simulink model "SEAMOUR_Sim"  (R2023a)
settings: Solver=ode4  StartTime=0.0  StopTime=12  FixedStep=simulation_ts  MaxStep=0.001  MinStep=0.0001  RelTol=1e-3  EnableMultiTasking=on
values from neighbouring files (symbols this model uses):
  Area_y = [0.0031581,0.024875,0.025026,0.021123,0.021123,0.025026,0.024875,0.037486]    [init_file.m]
  Area_z = [0.0031588,0.028932,0.035488,0.030129,0.030129,0.035488,0.028932,0.039984]    [init_file.m]
  Cd_y = [0.5645,0.5232,0.4085,0.3589,0.3589,0.40849,0.5232,0.4642]    [init_file.m]
  Cd_z = [0.5645,0.52,0.5843,0.533,0.533,0.5843,0.52,0.5238]    [init_file.m]
  Coeff = [xudot, yvdot, zwdot]    [init_file.m]
  gravity = 9.81    [init_file.m]
  m = (4*pi*rho*a*b*b)/3    (= 16.3133743522)    [init_file.m]
  offset = 0.002    [init_file.m]
  percent_y = Area_y/t_y    [init_file.m]
  percent_z = Area_z/t_z    [init_file.m]
  xudot = k1*m    [init_file.m]
undefined symbols (not defined in the file or in its folder): center_body, headmain, headmotorshield, headmount, hindconnection, hindcover, kx_lower, kx_upper, kz_lower, kz_upper, lefthindflipper, lefthindmotor, leftmotor1, leftmotor2, leftmotor3, lf_lower, lf_upper, rf_lower, rf_upper, righthindflipper, righthindmotor, rightmotor1, rightmotor2, rightmotor3, tailmotorshield, tailmount, X, Y, Z
libraries: nesl_utility x208, sm_lib x149
(part 5 of 7)

== system SEAMOUR_Sim/Sealion Robot/Distributed Forces/Distbuted Load In y and z directions/Subsystem1 ==
  Add10 : Sum
  Add11 : Sum
  Added Mass F : MATLAB Function  TreatAsAtomicUnit=on
  Body F : sm_lib/Frames and Transforms/Rigid Transform  TranslationMethod=Cartesian  TranslationStandardOffset=0  TranslationStandardOffsetUnits=m  TranslationStandardAxis=+Z  TranslationCartesianOffset=[0.09 0 0]  TranslationCartesianOffsetUnits=m  TranslationROffset=0  TranslationROffsetUnits=m  TranslationZOffset=0  TranslationZOffsetUnits=m  TranslationThetaOffset=0  TranslationThetaOffsetUnits=deg  RotationMethod=StandardAxis  RotationAngleUnits=deg  RotationStandardAxis=+X  RotationAngle=0  RotationArbitraryAxis=[0 0 1]  FollAlignAxisA=+X  BaseAlignAxisA=+Y  FollAlignAxisB=+Y  BaseAlignAxisB=+Z  RotationSequenceAxes=FollowerAxes  RotationSequence=XYX  RotationSequenceAngles=[0 0 0]  RotationSequenceAnglesUnits=deg  RotationMatrix=[1 0 0; 0 1 0; 0 0 1]  Quaternion=[1 0 0 0]
  Constant1 : Constant  Value=Cd_z
  Constant2 : Constant  Value=Area_z
  Constant25 : Constant  Value=Cd_y
  Constant26 : Constant  Value=Area_y
  Constant28 : Constant  Value=percent_y
  Constant29 : Constant  Value=Coeff
  Constant3 : Constant  Value=percent_z
  Drag F : MATLAB Function  TreatAsAtomicUnit=on
  External Force and Torque5 : sm_lib/Forces and Torques/External Force and Torque  ForceResolutionFrame=AttachedFrame  EnableForceX=off  EnableForceY=on  EnableForceZ=on  EnableForce=off  TorqueResolutionFrame=AttachedFrame  EnableTorqueX=off  EnableTorqueY=off  EnableTorqueZ=off  EnableTorque=off
  PS-Simulink Converter{28..29,42..43} (4 alike) : nesl_utility/PS-Simulink Converter  PhysicalDomain=network_engine_domain  SubClassName=ps_output  LeftPortType=input  RightPortType=output  PseudoPeriodic=off  Frequencies=[]  VectorFormat=1-D array  Unit=1  AffineConversion=off
  Scope : Scope
  Scope1 : Scope
  Simulink-PS Converter11 : nesl_utility/Simulink-PS Converter  PhysicalDomain=network_engine_domain  SubClassName=ps_input  LeftPortType=input  RightPortType=output  PseudoPeriodic=off  Frequencies=[]  NoiseDistribution=none  NoiseParameters=[]  Unit=1  AffineConversion=off  FilteringAndDerivatives=filter  SimscapeFilterOrder=2  InputFilterTimeConstant=0.001  UdotUserProvided=0
  Simulink-PS Converter12 : nesl_utility/Simulink-PS Converter  PhysicalDomain=network_engine_domain  SubClassName=ps_input  LeftPortType=input  RightPortType=output  PseudoPeriodic=off  Frequencies=[]  NoiseDistribution=none  NoiseParameters=[]  Unit=1  AffineConversion=off  FilteringAndDerivatives=filter  SimscapeFilterOrder=2  InputFilterTimeConstant=0.001  UdotUserProvided=0
  Transfer Fcn : TransferFcn  Denominator=[0.1 1]
  Transfer Fcn1 : TransferFcn  Denominator=[0.1 1]
  Transform Sensor5 : sm_lib/Frames and Transforms/Transform Sensor  MeasurementFrame=NonRotatingFollower  RotationSequence=XYX  SenseAngle=off  SenseAxis=off  SenseQ=off  SenseR=off  SenseRotationSequence=off  SenseOmegaX=off  SenseOmegaY=off  SenseOmegaZ=off  SenseQDot=off  SenseRDot=off  SenseRotationSequenceDot=off  SenseAlphaX=off  SenseAlphaY=off  SenseAlphaZ=off  SenseQDDot=off  SenseRDDot=off  SenseX=off  SenseY=off  SenseZ=off  SenseRad=off  SenseAzim=off  SenseDist=off  SenseInc=off  SenseXDot=off  SenseYDot=on  SenseZDot=on  SenseRadDot=off  SenseAzimDot=off  SenseDistDot=off  SenseIncDot=off  SenseXDDot=off  SenseYDDot=on  SenseZDDot=on  SenseRadDDot=off  SenseAzimDDot=off  SenseDistDDot=off  SenseIncDDot=off
  To CoM : PMIOPort  Side=Left
  To World Frame : PMIOPort  Port=2  Side=Left
  wires:
  Add10/1 -> Simulink-PS Converter11/1, Scope1/1
  PS-Simulink Converter29/1 -> Drag F/2(vel_z)  "Z"
  Constant28/1 -> Added Mass F/4(percent_y)
  Transfer Fcn1/1 -> Added Mass F/2(acc_z)
  PS-Simulink Converter43/1 -> Transfer Fcn1/1  "Z"
  Added Mass F/1(AM_Y) -> Add10/2
  Constant26/1 -> Drag F/5(Area_y)
  Drag F/2(D_Z) -> Add11/1
  PS-Simulink Converter42/1 -> Transfer Fcn/1  "Y"
  Constant25/1 -> Drag F/3(Cd_y)
  Constant1/1 -> Drag F/4(Cd_z)
  Constant29/1 -> Added Mass F/3(Coeff)
  Added Mass F/2(AM_Z) -> Add11/2
  PS-Simulink Converter28/1 -> Drag F/1(vel_y)  "Y"
  Drag F/1(D_Y) -> Add10/1
  Add11/1 -> Scope/1, Simulink-PS Converter12/1
  Constant3/1 -> Added Mass F/5(percent_z)
  Transfer Fcn/1 -> Added Mass F/1(acc_y)
  Constant2/1 -> Drag F/6(Area_z)
  connections:
  Body F/RConn1 -- Transform Sensor5/RConn1 -- External Force and Torque5/RConn1
  Body F/LConn1 -- To CoM/RConn1
  Transform Sensor5/RConn3 -- PS-Simulink Converter29/LConn1
  Transform Sensor5/RConn4 -- PS-Simulink Converter42/LConn1
  Transform Sensor5/RConn2 -- PS-Simulink Converter28/LConn1
  Simulink-PS Converter11/RConn1 -- External Force and Torque5/LConn1
  Transform Sensor5/LConn1 -- To World Frame/RConn1
  Transform Sensor5/RConn5 -- PS-Simulink Converter43/LConn1
  Simulink-PS Converter12/RConn1 -- External Force and Torque5/LConn2

== system SEAMOUR_Sim/Sealion Robot/Distributed Forces/Distbuted Load In y and z directions/Subsystem2 ==
  Add10 : Sum
  Add11 : Sum
  Added Mass F : MATLAB Function  TreatAsAtomicUnit=on
  Body F : sm_lib/Frames and Transforms/Rigid Transform  TranslationMethod=Cartesian  TranslationStandardOffset=0  TranslationStandardOffsetUnits=m  TranslationStandardAxis=+Z  TranslationCartesianOffset=[-0.02 0 0]  TranslationCartesianOffsetUnits=m  TranslationROffset=0  TranslationROffsetUnits=m  TranslationZOffset=0  TranslationZOffsetUnits=m  TranslationThetaOffset=0  TranslationThetaOffsetUnits=deg  RotationMethod=StandardAxis  RotationAngleUnits=deg  RotationStandardAxis=+X  RotationAngle=0  RotationArbitraryAxis=[0 0 1]  FollAlignAxisA=+X  BaseAlignAxisA=+Y  FollAlignAxisB=+Y  BaseAlignAxisB=+Z  RotationSequenceAxes=FollowerAxes  RotationSequence=XYX  RotationSequenceAngles=[0 0 0]  RotationSequenceAnglesUnits=deg  RotationMatrix=[1 0 0; 0 1 0; 0 0 1]  Quaternion=[1 0 0 0]
  Constant1 : Constant  Value=Cd_z
  Constant2 : Constant  Value=Area_z
  Constant25 : Constant  Value=Cd_y
  Constant26 : Constant  Value=Area_y
  Constant28 : Constant  Value=percent_y
  Constant29 : Constant  Value=Coeff
  Constant3 : Constant  Value=percent_z
  Drag F : MATLAB Function  TreatAsAtomicUnit=on
  External Force and Torque5 : sm_lib/Forces and Torques/External Force and Torque  ForceResolutionFrame=AttachedFrame  EnableForceX=off  EnableForceY=on  EnableForceZ=on  EnableForce=off  TorqueResolutionFrame=AttachedFrame  EnableTorqueX=off  EnableTorqueY=off  EnableTorqueZ=off  EnableTorque=off
  PS-Simulink Converter{28..29,42..43} (4 alike) : nesl_utility/PS-Simulink Converter  PhysicalDomain=network_engine_domain  SubClassName=ps_output  LeftPortType=input  RightPortType=output  PseudoPeriodic=off  Frequencies=[]  VectorFormat=1-D array  Unit=1  AffineConversion=off
  Scope : Scope
  Scope1 : Scope
  Simulink-PS Converter11 : nesl_utility/Simulink-PS Converter  PhysicalDomain=network_engine_domain  SubClassName=ps_input  LeftPortType=input  RightPortType=output  PseudoPeriodic=off  Frequencies=[]  NoiseDistribution=none  NoiseParameters=[]  Unit=1  AffineConversion=off  FilteringAndDerivatives=filter  SimscapeFilterOrder=2  InputFilterTimeConstant=0.001  UdotUserProvided=0
  Simulink-PS Converter12 : nesl_utility/Simulink-PS Converter  PhysicalDomain=network_engine_domain  SubClassName=ps_input  LeftPortType=input  RightPortType=output  PseudoPeriodic=off  Frequencies=[]  NoiseDistribution=none  NoiseParameters=[]  Unit=1  AffineConversion=off  FilteringAndDerivatives=filter  SimscapeFilterOrder=2  InputFilterTimeConstant=0.001  UdotUserProvided=0
  Transfer Fcn : TransferFcn  Denominator=[0.1 1]
  Transfer Fcn1 : TransferFcn  Denominator=[0.1 1]
  Transform Sensor5 : sm_lib/Frames and Transforms/Transform Sensor  MeasurementFrame=NonRotatingFollower  RotationSequence=XYX  SenseAngle=off  SenseAxis=off  SenseQ=off  SenseR=off  SenseRotationSequence=off  SenseOmegaX=off  SenseOmegaY=off  SenseOmegaZ=off  SenseQDot=off  SenseRDot=off  SenseRotationSequenceDot=off  SenseAlphaX=off  SenseAlphaY=off  SenseAlphaZ=off  SenseQDDot=off  SenseRDDot=off  SenseX=off  SenseY=off  SenseZ=off  SenseRad=off  SenseAzim=off  SenseDist=off  SenseInc=off  SenseXDot=off  SenseYDot=on  SenseZDot=on  SenseRadDot=off  SenseAzimDot=off  SenseDistDot=off  SenseIncDot=off  SenseXDDot=off  SenseYDDot=on  SenseZDDot=on  SenseRadDDot=off  SenseAzimDDot=off  SenseDistDDot=off  SenseIncDDot=off
  To CoM : PMIOPort  Side=Left
  To World Frame : PMIOPort  Port=2  Side=Left
  wires:
  Add10/1 -> Simulink-PS Converter11/1, Scope1/1
  PS-Simulink Converter29/1 -> Drag F/2(vel_z)  "Z"
  Constant28/1 -> Added Mass F/4(percent_y)
  Transfer Fcn1/1 -> Added Mass F/2(acc_z)
  PS-Simulink Converter43/1 -> Transfer Fcn1/1  "Z"
  Added Mass F/1(AM_Y) -> Add10/2
  Constant26/1 -> Drag F/5(Area_y)
  Drag F/2(D_Z) -> Add11/1
  PS-Simulink Converter42/1 -> Transfer Fcn/1  "Y"
  Constant25/1 -> Drag F/3(Cd_y)
  Constant1/1 -> Drag F/4(Cd_z)
  Constant29/1 -> Added Mass F/3(Coeff)
  Added Mass F/2(AM_Z) -> Add11/2
  PS-Simulink Converter28/1 -> Drag F/1(vel_y)  "Y"
  Drag F/1(D_Y) -> Add10/1
  Add11/1 -> Scope/1, Simulink-PS Converter12/1
  Constant3/1 -> Added Mass F/5(percent_z)
  Transfer Fcn/1 -> Added Mass F/1(acc_y)
  Constant2/1 -> Drag F/6(Area_z)
  connections:
  Body F/RConn1 -- Transform Sensor5/RConn1 -- External Force and Torque5/RConn1
  Body F/LConn1 -- To CoM/RConn1
  Transform Sensor5/RConn3 -- PS-Simulink Converter29/LConn1
  Transform Sensor5/RConn4 -- PS-Simulink Converter42/LConn1
  Transform Sensor5/RConn2 -- PS-Simulink Converter28/LConn1
  Simulink-PS Converter11/RConn1 -- External Force and Torque5/LConn1
  Transform Sensor5/LConn1 -- To World Frame/RConn1
  Transform Sensor5/RConn5 -- PS-Simulink Converter43/LConn1
  Simulink-PS Converter12/RConn1 -- External Force and Torque5/LConn2

== system SEAMOUR_Sim/Sealion Robot/Distributed Forces/Distbuted Load In y and z directions/Subsystem3 ==
  Add10 : Sum
  Add11 : Sum
  Added Mass F : MATLAB Function  TreatAsAtomicUnit=on
  Body F : sm_lib/Frames and Transforms/Rigid Transform  TranslationMethod=Cartesian  TranslationStandardOffset=0  TranslationStandardOffsetUnits=m  TranslationStandardAxis=+Z  TranslationCartesianOffset=[-0.1 0 0]  TranslationCartesianOffsetUnits=m  TranslationROffset=0  TranslationROffsetUnits=m  TranslationZOffset=0  TranslationZOffsetUnits=m  TranslationThetaOffset=0  TranslationThetaOffsetUnits=deg  RotationMethod=StandardAxis  RotationAngleUnits=deg  RotationStandardAxis=+X  RotationAngle=0  RotationArbitraryAxis=[0 0 1]  FollAlignAxisA=+X  BaseAlignAxisA=+Y  FollAlignAxisB=+Y  BaseAlignAxisB=+Z  RotationSequenceAxes=FollowerAxes  RotationSequence=XYX  RotationSequenceAngles=[0 0 0]  RotationSequenceAnglesUnits=deg  RotationMatrix=[1 0 0; 0 1 0; 0 0 1]  Quaternion=[1 0 0 0]
  Constant1 : Constant  Value=Cd_z
  Constant2 : Constant  Value=Area_z
  Constant25 : Constant  Value=Cd_y
  Constant26 : Constant  Value=Area_y
  Constant28 : Constant  Value=percent_y
  Constant29 : Constant  Value=Coeff
  Constant3 : Constant  Value=percent_z
  Drag F : MATLAB Function  TreatAsAtomicUnit=on
  External Force and Torque5 : sm_lib/Forces and Torques/External Force and Torque  ForceResolutionFrame=AttachedFrame  EnableForceX=off  EnableForceY=on  EnableForceZ=on  EnableForce=off  TorqueResolutionFrame=AttachedFrame  EnableTorqueX=off  EnableTorqueY=off  EnableTorqueZ=off  EnableTorque=off
  PS-Simulink Converter{28..29,42..43} (4 alike) : nesl_utility/PS-Simulink Converter  PhysicalDomain=network_engine_domain  SubClassName=ps_output  LeftPortType=input  RightPortType=output  PseudoPeriodic=off  Frequencies=[]  VectorFormat=1-D array  Unit=1  AffineConversion=off
  Scope : Scope
  Scope1 : Scope
  Simulink-PS Converter11 : nesl_utility/Simulink-PS Converter  PhysicalDomain=network_engine_domain  SubClassName=ps_input  LeftPortType=input  RightPortType=output  PseudoPeriodic=off  Frequencies=[]  NoiseDistribution=none  NoiseParameters=[]  Unit=1  AffineConversion=off  FilteringAndDerivatives=filter  SimscapeFilterOrder=2  InputFilterTimeConstant=0.001  UdotUserProvided=0
  Simulink-PS Converter12 : nesl_utility/Simulink-PS Converter  PhysicalDomain=network_engine_domain  SubClassName=ps_input  LeftPortType=input  RightPortType=output  PseudoPeriodic=off  Frequencies=[]  NoiseDistribution=none  NoiseParameters=[]  Unit=1  AffineConversion=off  FilteringAndDerivatives=filter  SimscapeFilterOrder=2  InputFilterTimeConstant=0.001  UdotUserProvided=0
  Transfer Fcn : TransferFcn  Denominator=[0.1 1]
  Transfer Fcn1 : TransferFcn  Denominator=[0.1 1]
  Transform Sensor5 : sm_lib/Frames and Transforms/Transform Sensor  MeasurementFrame=NonRotatingFollower  RotationSequence=XYX  SenseAngle=off  SenseAxis=off  SenseQ=off  SenseR=off  SenseRotationSequence=off  SenseOmegaX=off  SenseOmegaY=off  SenseOmegaZ=off  SenseQDot=off  SenseRDot=off  SenseRotationSequenceDot=off  SenseAlphaX=off  SenseAlphaY=off  SenseAlphaZ=off  SenseQDDot=off  SenseRDDot=off  SenseX=off  SenseY=off  SenseZ=off  SenseRad=off  SenseAzim=off  SenseDist=off  SenseInc=off  SenseXDot=off  SenseYDot=on  SenseZDot=on  SenseRadDot=off  SenseAzimDot=off  SenseDistDot=off  SenseIncDot=off  SenseXDDot=off  SenseYDDot=on  SenseZDDot=on  SenseRadDDot=off  SenseAzimDDot=off  SenseDistDDot=off  SenseIncDDot=off
  To CoM : PMIOPort  Side=Left
  To World Frame : PMIOPort  Port=2  Side=Left
  wires:
  Add10/1 -> Simulink-PS Converter11/1, Scope1/1
  PS-Simulink Converter29/1 -> Drag F/2(vel_z)  "Z"
  Constant28/1 -> Added Mass F/4(percent_y)
  Transfer Fcn1/1 -> Added Mass F/2(acc_z)
  PS-Simulink Converter43/1 -> Transfer Fcn1/1  "Z"
  Added Mass F/1(AM_Y) -> Add10/2
  Constant26/1 -> Drag F/5(Area_y)
  Drag F/2(D_Z) -> Add11/1
  PS-Simulink Converter42/1 -> Transfer Fcn/1  "Y"
  Constant25/1 -> Drag F/3(Cd_y)
  Constant1/1 -> Drag F/4(Cd_z)
  Constant29/1 -> Added Mass F/3(Coeff)
  Added Mass F/2(AM_Z) -> Add11/2
  PS-Simulink Converter28/1 -> Drag F/1(vel_y)  "Y"
  Drag F/1(D_Y) -> Add10/1
  Add11/1 -> Scope/1, Simulink-PS Converter12/1
  Constant3/1 -> Added Mass F/5(percent_z)
  Transfer Fcn/1 -> Added Mass F/1(acc_y)
  Constant2/1 -> Drag F/6(Area_z)
  connections:
  Body F/RConn1 -- Transform Sensor5/RConn1 -- External Force and Torque5/RConn1
  Body F/LConn1 -- To CoM/RConn1
  Transform Sensor5/RConn3 -- PS-Simulink Converter29/LConn1
  Transform Sensor5/RConn4 -- PS-Simulink Converter42/LConn1
  Transform Sensor5/RConn2 -- PS-Simulink Converter28/LConn1
  Simulink-PS Converter11/RConn1 -- External Force and Torque5/LConn1
  Transform Sensor5/LConn1 -- To World Frame/RConn1
  Transform Sensor5/RConn5 -- PS-Simulink Converter43/LConn1
  Simulink-PS Converter12/RConn1 -- External Force and Torque5/LConn2

== system SEAMOUR_Sim/Sealion Robot/Distributed Forces/Distbuted Load In y and z directions/Subsystem4 ==
  Add10 : Sum
  Add11 : Sum
  Added Mass F : MATLAB Function  TreatAsAtomicUnit=on
  Body F : sm_lib/Frames and Transforms/Rigid Transform  TranslationMethod=Cartesian  TranslationStandardOffset=0  TranslationStandardOffsetUnits=m  TranslationStandardAxis=+Z  TranslationCartesianOffset=[-0.185 0 0]  TranslationCartesianOffsetUnits=m  TranslationROffset=0  TranslationROffsetUnits=m  TranslationZOffset=0  TranslationZOffsetUnits=m  TranslationThetaOffset=0  TranslationThetaOffsetUnits=deg  RotationMethod=StandardAxis  RotationAngleUnits=deg  RotationStandardAxis=+X  RotationAngle=0  RotationArbitraryAxis=[0 0 1]  FollAlignAxisA=+X  BaseAlignAxisA=+Y  FollAlignAxisB=+Y  BaseAlignAxisB=+Z  RotationSequenceAxes=FollowerAxes  RotationSequence=XYX  RotationSequenceAngles=[0 0 0]  RotationSequenceAnglesUnits=deg  RotationMatrix=[1 0 0; 0 1 0; 0 0 1]  Quaternion=[1 0 0 0]
  Constant1 : Constant  Value=Cd_z
  Constant2 : Constant  Value=Area_z
  Constant25 : Constant  Value=Cd_y
  Constant26 : Constant  Value=Area_y
  Constant28 : Constant  Value=percent_y
  Constant29 : Constant  Value=Coeff
  Constant3 : Constant  Value=percent_z
  Drag F : MATLAB Function  TreatAsAtomicUnit=on
  External Force and Torque5 : sm_lib/Forces and Torques/External Force and Torque  ForceResolutionFrame=AttachedFrame  EnableForceX=off  EnableForceY=on  EnableForceZ=on  EnableForce=off  TorqueResolutionFrame=AttachedFrame  EnableTorqueX=off  EnableTorqueY=off  EnableTorqueZ=off  EnableTorque=off
  PS-Simulink Converter{1..2,28..29} (4 alike) : nesl_utility/PS-Simulink Converter  PhysicalDomain=network_engine_domain  SubClassName=ps_output  LeftPortType=input  RightPortType=output  PseudoPeriodic=off  Frequencies=[]  VectorFormat=1-D array  Unit=1  AffineConversion=off
  Scope : Scope
  Scope1 : Scope
  Simulink-PS Converter11 : nesl_utility/Simulink-PS Converter  PhysicalDomain=network_engine_domain  SubClassName=ps_input  LeftPortType=input  RightPortType=output  PseudoPeriodic=off  Frequencies=[]  NoiseDistribution=none  NoiseParameters=[]  Unit=1  AffineConversion=off  FilteringAndDerivatives=filter  SimscapeFilterOrder=2  InputFilterTimeConstant=0.001  UdotUserProvided=0
  Simulink-PS Converter12 : nesl_utility/Simulink-PS Converter  PhysicalDomain=network_engine_domain  SubClassName=ps_input  LeftPortType=input  RightPortType=output  PseudoPeriodic=off  Frequencies=[]  NoiseDistribution=none  NoiseParameters=[]  Unit=1  AffineConversion=off  FilteringAndDerivatives=filter  SimscapeFilterOrder=2  InputFilterTimeConstant=0.001  UdotUserProvided=0
  Transfer Fcn2 : TransferFcn  Denominator=[0.1 1]
  Transfer Fcn3 : TransferFcn  Denominator=[0.1 1]
  Transform Sensor5 : sm_lib/Frames and Transforms/Transform Sensor  MeasurementFrame=NonRotatingFollower  RotationSequence=XYX  SenseAngle=off  SenseAxis=off  SenseQ=off  SenseR=off  SenseRotationSequence=off  SenseOmegaX=off  SenseOmegaY=off  SenseOmegaZ=off  SenseQDot=off  SenseRDot=off  SenseRotationSequenceDot=off  SenseAlphaX=off  SenseAlphaY=off  SenseAlphaZ=off  SenseQDDot=off  SenseRDDot=off  SenseX=off  SenseY=off  SenseZ=off  SenseRad=off  SenseAzim=off  SenseDist=off  SenseInc=off  SenseXDot=off  SenseYDot=on  SenseZDot=on  SenseRadDot=off  SenseAzimDot=off  SenseDistDot=off  SenseIncDot=off  SenseXDDot=off  SenseYDDot=on  SenseZDDot=on  SenseRadDDot=off  SenseAzimDDot=off  SenseDistDDot=off  SenseIncDDot=off
  To CoM : PMIOPort  Side=Left
  To World Frame : PMIOPort  Port=2  Side=Left
  wires:
  Add10/1 -> Simulink-PS Converter11/1, Scope1/1
  PS-Simulink Converter29/1 -> Drag F/2(vel_z)  "Z"
  Constant28/1 -> Added Mass F/4(percent_y)
  Transfer Fcn3/1 -> Added Mass F/2(acc_z)
  PS-Simulink Converter2/1 -> Transfer Fcn3/1  "Z"
  Added Mass F/1(AM_Y) -> Add10/2
  Constant26/1 -> Drag F/5(Area_y)
  Drag F/2(D_Z) -> Add11/1
  PS-Simulink Converter1/1 -> Transfer Fcn2/1  "Y"
  Constant25/1 -> Drag F/3(Cd_y)
  Constant1/1 -> Drag F/4(Cd_z)
  Constant29/1 -> Added Mass F/3(Coeff)
  Added Mass F/2(AM_Z) -> Add11/2
  PS-Simulink Converter28/1 -> Drag F/1(vel_y)  "Y"
  Drag F/1(D_Y) -> Add10/1
  Add11/1 -> Scope/1, Simulink-PS Converter12/1
  Constant3/1 -> Added Mass F/5(percent_z)
  Transfer Fcn2/1 -> Added Mass F/1(acc_y)
  Constant2/1 -> Drag F/6(Area_z)
  connections:
  Body F/RConn1 -- Transform Sensor5/RConn1 -- External Force and Torque5/RConn1
  Body F/LConn1 -- To CoM/RConn1
  Transform Sensor5/RConn2 -- PS-Simulink Converter28/LConn1
  Simulink-PS Converter12/RConn1 -- External Force and Torque5/LConn2
  Transform Sensor5/RConn3 -- PS-Simulink Converter29/LConn1
  Transform Sensor5/LConn1 -- To World Frame/RConn1
  Transform Sensor5/RConn4 -- PS-Simulink Converter1/LConn1
  Simulink-PS Converter11/RConn1 -- External Force and Torque5/LConn1
  Transform Sensor5/RConn5 -- PS-Simulink Converter2/LConn1

== system SEAMOUR_Sim/Sealion Robot/Distributed Forces/Distbuted Load In y and z directions/Subsystem5 ==
  Add10 : Sum
  Add11 : Sum
  Added Mass F : MATLAB Function  TreatAsAtomicUnit=on
  Body F : sm_lib/Frames and Transforms/Rigid Transform  TranslationMethod=Cartesian  TranslationStandardOffset=0  TranslationStandardOffsetUnits=m  TranslationStandardAxis=+Z  TranslationCartesianOffset=[-0.265 0 0]  TranslationCartesianOffsetUnits=m  TranslationROffset=0  TranslationROffsetUnits=m  TranslationZOffset=0  TranslationZOffsetUnits=m  TranslationThetaOffset=0  TranslationThetaOffsetUnits=deg  RotationMethod=StandardAxis  RotationAngleUnits=deg  RotationStandardAxis=+X  RotationAngle=0  RotationArbitraryAxis=[0 0 1]  FollAlignAxisA=+X  BaseAlignAxisA=+Y  FollAlignAxisB=+Y  BaseAlignAxisB=+Z  RotationSequenceAxes=FollowerAxes  RotationSequence=XYX  RotationSequenceAngles=[0 0 0]  RotationSequenceAnglesUnits=deg  RotationMatrix=[1 0 0; 0 1 0; 0 0 1]  Quaternion=[1 0 0 0]
  Constant1 : Constant  Value=Cd_z
  Constant2 : Constant  Value=Area_z
  Constant25 : Constant  Value=Cd_y
  Constant26 : Constant  Value=Area_y
  Constant28 : Constant  Value=percent_y
  Constant29 : Constant  Value=Coeff
  Constant3 : Constant  Value=percent_z
  Drag F : MATLAB Function  TreatAsAtomicUnit=on
  External Force and Torque5 : sm_lib/Forces and Torques/External Force and Torque  ForceResolutionFrame=AttachedFrame  EnableForceX=off  EnableForceY=on  EnableForceZ=on  EnableForce=off  TorqueResolutionFrame=AttachedFrame  EnableTorqueX=off  EnableTorqueY=off  EnableTorqueZ=off  EnableTorque=off
  PS-Simulink Converter{28..29,42..43} (4 alike) : nesl_utility/PS-Simulink Converter  PhysicalDomain=network_engine_domain  SubClassName=ps_output  LeftPortType=input  RightPortType=output  PseudoPeriodic=off  Frequencies=[]  VectorFormat=1-D array  Unit=1  AffineConversion=off
  Scope : Scope
  Scope1 : Scope
  Simulink-PS Converter11 : nesl_utility/Simulink-PS Converter  PhysicalDomain=network_engine_domain  SubClassName=ps_input  LeftPortType=input  RightPortType=output  PseudoPeriodic=off  Frequencies=[]  NoiseDistribution=none  NoiseParameters=[]  Unit=1  AffineConversion=off  FilteringAndDerivatives=filter  SimscapeFilterOrder=2  InputFilterTimeConstant=0.001  UdotUserProvided=0
  Simulink-PS Converter12 : nesl_utility/Simulink-PS Converter  PhysicalDomain=network_engine_domain  SubClassName=ps_input  LeftPortType=input  RightPortType=output  PseudoPeriodic=off  Frequencies=[]  NoiseDistribution=none  NoiseParameters=[]  Unit=1  AffineConversion=off  FilteringAndDerivatives=filter  SimscapeFilterOrder=2  InputFilterTimeConstant=0.001  UdotUserProvided=0
  Transfer Fcn : TransferFcn  Denominator=[0.1 1]
  Transfer Fcn1 : TransferFcn  Denominator=[0.1 1]
  Transform Sensor5 : sm_lib/Frames and Transforms/Transform Sensor  MeasurementFrame=NonRotatingFollower  RotationSequence=XYX  SenseAngle=off  SenseAxis=off  SenseQ=off  SenseR=off  SenseRotationSequence=off  SenseOmegaX=off  SenseOmegaY=off  SenseOmegaZ=off  SenseQDot=off  SenseRDot=off  SenseRotationSequenceDot=off  SenseAlphaX=off  SenseAlphaY=off  SenseAlphaZ=off  SenseQDDot=off  SenseRDDot=off  SenseX=off  SenseY=off  SenseZ=off  SenseRad=off  SenseAzim=off  SenseDist=off  SenseInc=off  SenseXDot=off  SenseYDot=on  SenseZDot=on  SenseRadDot=off  SenseAzimDot=off  SenseDistDot=off  SenseIncDot=off  SenseXDDot=off  SenseYDDot=on  SenseZDDot=on  SenseRadDDot=off  SenseAzimDDot=off  SenseDistDDot=off  SenseIncDDot=off
  To CoM : PMIOPort  Side=Left
  To World Frame : PMIOPort  Port=2  Side=Left
  wires:
  Constant28/1 -> Added Mass F/4(percent_y)
  PS-Simulink Converter29/1 -> Drag F/2(vel_z)  "Z"
  Added Mass F/1(AM_Y) -> Add10/2
  Add10/1 -> Simulink-PS Converter11/1, Scope1/1
  Constant26/1 -> Drag F/5(Area_y)
  Constant25/1 -> Drag F/3(Cd_y)
  Drag F/2(D_Z) -> Add11/1
  Add11/1 -> Scope/1, Simulink-PS Converter12/1
  Added Mass F/2(AM_Z) -> Add11/2
  PS-Simulink Converter28/1 -> Drag F/1(vel_y)  "Y"
  Constant29/1 -> Added Mass F/3(Coeff)
  Drag F/1(D_Y) -> Add10/1
  PS-Simulink Converter42/1 -> Transfer Fcn/1  "Y"
  Transfer Fcn/1 -> Added Mass F/1(acc_y)
  PS-Simulink Converter43/1 -> Transfer Fcn1/1  "Z"
  Transfer Fcn1/1 -> Added Mass F/2(acc_z)
  Constant1/1 -> Drag F/4(Cd_z)
  Constant2/1 -> Drag F/6(Area_z)
  Constant3/1 -> Added Mass F/5(percent_z)
  connections:
  Simulink-PS Converter11/RConn1 -- External Force and Torque5/LConn1
  Simulink-PS Converter12/RConn1 -- External Force and Torque5/LConn2
  Transform Sensor5/RConn3 -- PS-Simulink Converter29/LConn1
  Transform Sensor5/RConn2 -- PS-Simulink Converter28/LConn1
  External Force and Torque5/RConn1 -- Transform Sensor5/RConn1 -- Body F/RConn1
  Transform Sensor5/LConn1 -- To World Frame/RConn1
  Body F/LConn1 -- To CoM/RConn1
  Transform Sensor5/RConn5 -- PS-Simulink Converter43/LConn1
  Transform Sensor5/RConn4 -- PS-Simulink Converter42/LConn1

== system SEAMOUR_Sim/Sealion Robot/HEAD/Head/Subsystem ==
  Add10 : Sum
  Add11 : Sum
  Added Mass F : MATLAB Function  TreatAsAtomicUnit=on
  Constant2 : Constant
  Constant25 : Constant  Value=Cd_y
  Constant26 : Constant  Value=Area_y
  Constant28 : Constant  Value=percent_y
  Constant29 : Constant  Value=Coeff
  Constant3 : Constant  Value=Cd_z
  Constant4 : Constant  Value=Area_z
  Constant5 : Constant  Value=percent_z
  Drag F : MATLAB Function  TreatAsAtomicUnit=on
  External Force and Torque5 : sm_lib/Forces and Torques/External Force and Torque  ForceResolutionFrame=AttachedFrame  EnableForceX=off  EnableForceY=on  EnableForceZ=on  EnableForce=off  TorqueResolutionFrame=AttachedFrame  EnableTorqueX=off  EnableTorqueY=off  EnableTorqueZ=off  EnableTorque=off
  PS-Simulink Converter{28..29,42..43} (4 alike) : nesl_utility/PS-Simulink Converter  PhysicalDomain=network_engine_domain  SubClassName=ps_output  LeftPortType=input  RightPortType=output  PseudoPeriodic=off  Frequencies=[]  VectorFormat=1-D array  Unit=1  AffineConversion=off
  Scope : Scope
  Scope1 : Scope
  Simulink-PS Converter11 : nesl_utility/Simulink-PS Converter  PhysicalDomain=network_engine_domain  SubClassName=ps_input  LeftPortType=input  RightPortType=output  PseudoPeriodic=off  Frequencies=[]  NoiseDistribution=none  NoiseParameters=[]  Unit=1  AffineConversion=off  FilteringAndDerivatives=filter  SimscapeFilterOrder=2  InputFilterTimeConstant=0.001  UdotUserProvided=0
  Simulink-PS Converter12 : nesl_utility/Simulink-PS Converter  PhysicalDomain=network_engine_domain  SubClassName=ps_input  LeftPortType=input  RightPortType=output  PseudoPeriodic=off  Frequencies=[]  NoiseDistribution=none  NoiseParameters=[]  Unit=1  AffineConversion=off  FilteringAndDerivatives=filter  SimscapeFilterOrder=2  InputFilterTimeConstant=0.001  UdotUserProvided=0
  Transfer Fcn : TransferFcn  Denominator=[0.1 1]
  Transfer Fcn1 : TransferFcn  Denominator=[0.1 1]
  Transform Sensor5 : sm_lib/Frames and Transforms/Transform Sensor  MeasurementFrame=NonRotatingFollower  RotationSequence=XYX  SenseAngle=off  SenseAxis=off  SenseQ=off  SenseR=off  SenseRotationSequence=off  SenseOmegaX=off  SenseOmegaY=off  SenseOmegaZ=off  SenseQDot=off  SenseRDot=off  SenseRotationSequenceDot=off  SenseAlphaX=off  SenseAlphaY=off  SenseAlphaZ=off  SenseQDDot=off  SenseRDDot=off  SenseX=off  SenseY=off  SenseZ=off  SenseRad=off  SenseAzim=off  SenseDist=off  SenseInc=off  SenseXDot=off  SenseYDot=on  SenseZDot=on  SenseRadDot=off  SenseAzimDot=off  SenseDistDot=off  SenseIncDot=off  SenseXDDot=off  SenseYDDot=on  SenseZDDot=on  SenseRadDDot=off  SenseAzimDDot=off  SenseDistDDot=off  SenseIncDDot=off
  To Head : PMIOPort  Side=Left
  To World frame : PMIOPort  Port=2  Side=Left
  wires:
  PS-Simulink Converter43/1 -> Transfer Fcn1/1  "Z"
  Constant25/1 -> Drag F/3(Cd_y)
  Drag F/1(D_Y) -> Add10/1
  Constant2/1 -> Drag F/7(scale)
  PS-Simulink Converter28/1 -> Drag F/1(vel_y)  "Y"
  Add11/1 -> Scope/1, Simulink-PS Converter12/1
  Transfer Fcn1/1 -> Added Mass F/2(acc_z)
  Constant5/1 -> Added Mass F/5(percent_z)
  Drag F/2(D_Z) -> Add11/1
  Added Mass F/2(AM_Z) -> Add11/2
  Add10/1 -> Simulink-PS Converter11/1, Scope1/1
  Constant28/1 -> Added Mass F/4(percent_y)
  Constant26/1 -> Drag F/5(Area_y)
  Constant4/1 -> Drag F/6(Area_z)
  Added Mass F/1(AM_Y) -> Add10/2
  PS-Simulink Converter42/1 -> Transfer Fcn/1  "Y"
  Constant29/1 -> Added Mass F/3(Coeff)
  PS-Simulink Converter29/1 -> Drag F/2(vel_z)  "Z"
  Constant3/1 -> Drag F/4(Cd_z)
  Transfer Fcn/1 -> Added Mass F/1(acc_y)
  connections:
  External Force and Torque5/RConn1 -- To Head/RConn1 -- Transform Sensor5/RConn1
  Transform Sensor5/RConn5 -- PS-Simulink Converter43/LConn1
  Simulink-PS Converter11/RConn1 -- External Force and Torque5/LConn1
  Transform Sensor5/RConn3 -- PS-Simulink Converter29/LConn1
  Transform Sensor5/RConn4 -- PS-Simulink Converter42/LConn1
  Transform Sensor5/RConn2 -- PS-Simulink Converter28/LConn1
  Transform Sensor5/LConn1 -- To World frame/RConn1
  Simulink-PS Converter12/RConn1 -- External Force and Torque5/LConn2

== system SEAMOUR_Sim/Sealion Robot/LEFT FLIPPER/Left Motors/MOTOR 1 ==
  Left Motor 1 : sm_lib/Body Elements/File Solid  ExtGeomFileName=Simscape_Parts_StepFiles/motor_1_left_mirror.stp  UnitType=FromFile  ExtGeomFileUnits=m  StepReaderType=HEX  ExportConvexHullGeometry=off  InertiaType=Custom  Mass=leftmotor1.mass  MassUnits=kg  CenterOfMass=leftmotor1.com  CenterOfMassUnits=m  MomentsOfInertia=leftmotor1.inertia  MomentsOfInertiaUnits=kg*m^2  ProductsOfInertia=leftmotor1.prodinertia  ProductsOfInertiaUnits=kg*m^2  BasedOnType=Density  Density=2.7  DensityUnits=g/cm^3  DoExposeReferenceFrame=off  SerializedFrames=<Frames><Frame><Id>Frame1</Id><Value><Name>CoM</Name><Origin><Source>CenterOfMassFrame</Source><FeatureName></FeatureName></Origin><PrimaryAxis><DefinedDirection>-Z</DefinedDirection><Source>GeometricFeature</Source><SourceDirection>+Z</SourceDirection><FeatureName>planar surface 14</FeatureName></PrimaryAxis><SecondaryAxis><DefinedDirection>+X</DefinedDirection><Source>GeometricFeature</Source><SourceDirection>+X</SourceDirection><FeatureName>planar surface 10</FeatureName></SecondaryAxis></Value></Frame><Frame><Id>Frame2</Id><Value><Name>To Center</Name><Origin><Source>GeometricFeature</Source><FeatureName>circular curve 1</FeatureName></Origin><PrimaryAxis><DefinedDirection>+Z</DefinedDirection><Source>ReferenceFrame</Source><SourceDirection>+Y</SourceDirection><FeatureName></FeatureName></PrimaryAxis><SecondaryAxis><DefinedDirection>-Y</DefinedDirection><Source>ReferenceFrame</Source><SourceDirection>+X</SourceDirection><FeatureName></FeatureName></SecondaryAxis></Value></Frame><Frame><Id>Frame3</Id><Value><Name>To Motor 2</Name><Origin><Source>GeometricFeature</Source><FeatureName>circular curve 528</FeatureName></Origin><PrimaryAxis><DefinedDirection>+X</DefinedDirection><Source>ReferenceFrame</Source><SourceDirection>+Z</SourceDirection><FeatureName></FeatureName></PrimaryAxis><SecondaryAxis><DefinedDirection>-Y</DefinedDirection><Source>ReferenceFrame</Source><SourceDirection>+Y</SourceDirection><FeatureName></FeatureName></SecondaryAxis></Value></Frame></Frames>  GraphicType=FromGeometry  MarkerShape=Sphere  MarkerSize=10  GraphicVisPropType=SimpleVisualProperties  GraphicDiffuseColor=[0.6 0.0 0.0]  GraphicSpecularColor=[0.5 0.5 0.5 1.0]  GraphicAmbientColor=[0.15 0.15 0.15 1.0]  GraphicEmissiveColor=[0.0 0.0 0.0 1.0]  GraphicShininess=75  GraphicOpacity=1.0
  Mux : Mux  Inputs=3
  PS-Simulink Converter1 : nesl_utility/PS-Simulink Converter  PhysicalDomain=network_engine_domain  SubClassName=ps_output  LeftPortType=input  RightPortType=output  PseudoPeriodic=off  Frequencies=[]  VectorFormat=1-D array  Unit=1  AffineConversion=off
  PS-Simulink Converter12 : nesl_utility/PS-Simulink Converter  PhysicalDomain=network_engine_domain  SubClassName=ps_output  LeftPortType=input  RightPortType=output  PseudoPeriodic=off  Frequencies=[]  VectorFormat=1-D array  Unit=1  AffineConversion=off
  PS-Simulink Converter2 : nesl_utility/PS-Simulink Converter  PhysicalDomain=network_engine_domain  SubClassName=ps_output  LeftPortType=input  RightPortType=output  PseudoPeriodic=off  Frequencies=[]  VectorFormat=1-D array  Unit=1  AffineConversion=off
  Rigid Transform : sm_lib/Frames and Transforms/Rigid Transform  TranslationMethod=Cartesian  TranslationStandardOffset=0  TranslationStandardOffsetUnits=mm  TranslationStandardAxis=+Z  TranslationCartesianOffset=[0 0 0]  TranslationCartesianOffsetUnits=mm  TranslationROffset=0  TranslationROffsetUnits=m  TranslationZOffset=0  TranslationZOffsetUnits=m  TranslationThetaOffset=0  TranslationThetaOffsetUnits=deg  RotationMethod=StandardAxis  RotationAngleUnits=deg  RotationStandardAxis=+X  RotationAngle=180  RotationArbitraryAxis=[0 0 1]  FollAlignAxisA=+X  BaseAlignAxisA=+Y  FollAlignAxisB=+Y  BaseAlignAxisB=+Z  RotationSequenceAxes=FollowerAxes  RotationSequence=XYX  RotationSequenceAngles=[0 0 0]  RotationSequenceAnglesUnits=deg  RotationMatrix=[1 0 0; 0 1 0; 0 0 1]  Quaternion=[1 0 0 0]
  Rigid Transform1 : sm_lib/Frames and Transforms/Rigid Transform  TranslationMethod=Cartesian  TranslationStandardOffset=0  TranslationStandardOffsetUnits=mm  TranslationStandardAxis=+Z  TranslationCartesianOffset=[0 0 0]  TranslationCartesianOffsetUnits=mm  TranslationROffset=0  TranslationROffsetUnits=m  TranslationZOffset=0  TranslationZOffsetUnits=m  TranslationThetaOffset=0  TranslationThetaOffsetUnits=deg  RotationMethod=StandardAxis  RotationAngleUnits=deg  RotationStandardAxis=+Z  RotationAngle=180  RotationArbitraryAxis=[0 0 1]  FollAlignAxisA=+X  BaseAlignAxisA=+Y  FollAlignAxisB=+Y  BaseAlignAxisB=+Z  RotationSequenceAxes=FollowerAxes  RotationSequence=XYX  RotationSequenceAngles=[0 0 0]  RotationSequenceAnglesUnits=deg  RotationMatrix=[1 0 0; 0 1 0; 0 0 1]  Quaternion=[1 0 0 0]
  Rigid Transform4 : sm_lib/Frames and Transforms/Rigid Transform  TranslationMethod=Cartesian  TranslationStandardOffset=0  TranslationStandardOffsetUnits=mm  TranslationStandardAxis=+Z  TranslationCartesianOffset=[0 0 0]  TranslationCartesianOffsetUnits=mm  TranslationROffset=0  TranslationROffsetUnits=m  TranslationZOffset=0  TranslationZOffsetUnits=m  TranslationThetaOffset=0  TranslationThetaOffsetUnits=deg  RotationMethod=StandardAxis  RotationAngleUnits=deg  RotationStandardAxis=+Y  RotationAngle=0  RotationArbitraryAxis=[0 0 1]  FollAlignAxisA=+X  BaseAlignAxisA=+Y  FollAlignAxisB=+Y  BaseAlignAxisB=+Z  RotationSequenceAxes=FollowerAxes  RotationSequence=XYX  RotationSequenceAngles=[0 0 0]  RotationSequenceAnglesUnits=deg  RotationMatrix=[1 0 0; 0 1 0; 0 0 1]  Quaternion=[1 0 0 0]
  To Workspace : ToWorkspace  VariableName=left_motor1  SampleTime=-1
      settings: Save2DSignal=2-D array (concatenate along first dimension)
  Transform Sensor3 : sm_lib/Frames and Transforms/Transform Sensor  MeasurementFrame=NonRotatingFollower  RotationSequence=XYX  SenseAngle=off  SenseAxis=off  SenseQ=off  SenseR=off  SenseRotationSequence=off  SenseOmegaX=off  SenseOmegaY=off  SenseOmegaZ=off  SenseQDot=off  SenseRDot=off  SenseRotationSequenceDot=off  SenseAlphaX=off  SenseAlphaY=off  SenseAlphaZ=off  SenseQDDot=off  SenseRDDot=off  SenseX=on  SenseY=on  SenseZ=on  SenseRad=off  SenseAzim=off  SenseDist=off  SenseInc=off  SenseXDot=off  SenseYDot=off  SenseZDot=off  SenseRadDot=off  SenseAzimDot=off  SenseDistDot=off  SenseIncDot=off  SenseXDDot=off  SenseYDDot=off  SenseZDDot=off  SenseRadDDot=off  SenseAzimDDot=off  SenseDistDDot=off  SenseIncDDot=off
  To Center : PMIOPort  Side=Left
  To Motor 2 : PMIOPort  Port=2  Side=Right
  World Frame : PMIOPort  Port=3  Side=Right
  tag scope: left_motor1=global
  wires:
  PS-Simulink Converter1/1 -> Mux/2  "y"
  PS-Simulink Converter12/1 -> Mux/1  "x"
  Mux/1 -> [left_motor1], To Workspace/1
  PS-Simulink Converter2/1 -> Mux/3  "z"
  connections:
  Rigid Transform/RConn1 -- Rigid Transform4/LConn1
  Left Motor 1/LConn2 -- Transform Sensor3/RConn1 -- To Motor 2/RConn1
  Rigid Transform1/RConn1 -- Left Motor 1/RConn1
  To Center/RConn1 -- Rigid Transform/LConn1
  Rigid Transform4/RConn1 -- Rigid Transform1/LConn1
  PS-Simulink Converter2/LConn1 -- Transform Sensor3/RConn4
  PS-Simulink Converter12/LConn1 -- Transform Sensor3/RConn2
  PS-Simulink Converter1/LConn1 -- Transform Sensor3/RConn3
  World Frame/RConn1 -- Transform Sensor3/LConn1

== system SEAMOUR_Sim/Sealion Robot/LEFT FLIPPER/Left Motors/MOTOR 2 ==
  Left Motor 2 : sm_lib/Body Elements/File Solid  ExtGeomFileName=Simscape_Parts_StepFiles/motor_2_left.stp  UnitType=FromFile  ExtGeomFileUnits=m  StepReaderType=HEX  ExportConvexHullGeometry=off  InertiaType=Custom  Mass=leftmotor2.mass  MassUnits=kg  CenterOfMass=leftmotor2.com  CenterOfMassUnits=m  MomentsOfInertia=leftmotor2.inertia  MomentsOfInertiaUnits=kg*m^2  ProductsOfInertia=leftmotor2.prodinertia  ProductsOfInertiaUnits=kg*m^2  BasedOnType=Density  Density=2.7  DensityUnits=g/cm^3  DoExposeReferenceFrame=off  SerializedFrames=<Frames><Frame><Id>Frame2</Id><Value><Name>To motor 1</Name><Origin><Source>GeometricFeature</Source><FeatureName>circular curve 1185</FeatureName></Origin><PrimaryAxis><DefinedDirection>+Z</DefinedDirection><Source>GeometricFeature</Source><SourceDirection>+Z</SourceDirection><FeatureName>circular curve 2</FeatureName></PrimaryAxis><SecondaryAxis><DefinedDirection>-Y</DefinedDirection><Source>GeometricFeature</Source><SourceDirection>+X</SourceDirection><FeatureName>segment 1823</FeatureName></SecondaryAxis></Value></Frame><Frame><Id>Frame3</Id><Value><Name>To Motor 3</Name><Origin><Source>GeometricFeature</Source><FeatureName>circular curve 971</FeatureName></Origin><PrimaryAxis><DefinedDirection>+Y</DefinedDirection><Source>GeometricFeature</Source><SourceDirection>+Z</SourceDirection><FeatureName>segment 29</FeatureName></PrimaryAxis><SecondaryAxis><DefinedDirection>+X</DefinedDirection><Source>GeometricFeature</Source><SourceDirection>+X</SourceDirection><FeatureName>segment 10</FeatureName></SecondaryAxis></Value></Frame><Frame><Id>Frame4</Id><Value><Name>COM</Name><Origin><Source>CenterOfMassFrame</Source><FeatureName></FeatureName></Origin><PrimaryAxis><DefinedDirection>-X</DefinedDirection><Source>GeometricFeature</Source><SourceDirection>+Z</SourceDirection><FeatureName>planar surface 3</FeatureName></PrimaryAxis><SecondaryAxis><DefinedDirection>-Y</DefinedDirection><Source>GeometricFeature</Source><SourceDirection>+X</SourceDirection><FeatureName>planar surface 273</FeatureName></SecondaryAxis></Value></Frame></Frames>  GraphicType=FromGeometry  MarkerShape=Sphere  MarkerSize=10  GraphicVisPropType=SimpleVisualProperties  GraphicDiffuseColor=[1.0 0.2 0.2]  GraphicSpecularColor=[0.5 0.5 0.5 1.0]  GraphicAmbientColor=[0.15 0.15 0.15 1.0]  GraphicEmissiveColor=[0.0 0.0 0.0 1.0]  GraphicShininess=75  GraphicOpacity=1.0
  Mux : Mux  Inputs=3
  PS-Simulink Converter : nesl_utility/PS-Simulink Converter  PhysicalDomain=network_engine_domain  SubClassName=ps_output  LeftPortType=input  RightPortType=output  PseudoPeriodic=off  Frequencies=[]  VectorFormat=inherit  Unit=inherit  AffineConversion=off
  PS-Simulink Converter12 : nesl_utility/PS-Simulink Converter  PhysicalDomain=network_engine_domain  SubClassName=ps_output  LeftPortType=input  RightPortType=output  PseudoPeriodic=off  Frequencies=[]  VectorFormat=1-D array  Unit=1  AffineConversion=off
  PS-Simulink Converter2 : nesl_utility/PS-Simulink Converter  PhysicalDomain=network_engine_domain  SubClassName=ps_output  LeftPortType=input  RightPortType=output  PseudoPeriodic=off  Frequencies=[]  VectorFormat=1-D array  Unit=1  AffineConversion=off
  PS-Simulink Converter3 : nesl_utility/PS-Simulink Converter  PhysicalDomain=network_engine_domain  SubClassName=ps_output  LeftPortType=input  RightPortType=output  PseudoPeriodic=off  Frequencies=[]  VectorFormat=1-D array  Unit=1  AffineConversion=off
  PS-Simulink Converter4 : nesl_utility/PS-Simulink Converter  PhysicalDomain=network_engine_domain  SubClassName=ps_output  LeftPortType=input  RightPortType=output  PseudoPeriodic=off  Frequencies=[]  VectorFormat=inherit  Unit=inherit  AffineConversion=off
  PS-Simulink Converter6 : nesl_utility/PS-Simulink Converter  PhysicalDomain=network_engine_domain  SubClassName=ps_output  LeftPortType=input  RightPortType=output  PseudoPeriodic=off  Frequencies=[]  VectorFormat=inherit  Unit=inherit  AffineConversion=off
  Product : Product
  Revolute Joint : sm_lib/Joints/Revolute Joint  JointMode=Normal  SenseConstraintForce=off  SenseConstraintForceX=off  SenseConstraintForceY=off  SenseConstraintForceZ=off  SenseConstraintTorque=off  SenseConstraintTorqueX=off  SenseConstraintTorqueY=off  SenseConstraintTorqueZ=off  SenseTotalForce=off  SenseTotalForceX=off  SenseTotalForceY=off  SenseTotalForceZ=off  SenseTotalTorque=off  SenseTotalTorqueX=off  SenseTotalTorqueY=off  SenseTotalTorqueZ=off  CompositeWrenchDir=FollowerOnBase  CompositeWrenchFrame=BaseFrame  EquilibriumPosition=0  EquilibriumPositionUnits=deg  SpringStiffness=0  SpringStiffnessUnits=N*m/deg  DampingCoefficient=0  DampingCoefficientUnits=N*m/(deg/s)  TorqueActuationMode=ComputedTorque  MotionActuationMode=InputMotion  SensePosition=on  SenseVelocity=on  SenseAcceleration=off  SenseTorqueForce=on  SenseLowerLimitTorqueForce=off  SenseUpperLimitTorqueForce=off  LowerLimitSpecify=off  LowerLimitBound=-90  LowerLimitBoundUnits=deg  LowerLimitStiffness=1e4  LowerLimitStiffnessUnits=N*m/deg  LowerLimitDamping=10  LowerLimitDampingUnits=N*m/(deg/s)  LowerLimitTransitionRegionWidth=0.1  LowerLimitTransitionRegionWidthUnits=deg  UpperLimitSpecify=off  UpperLimitBound=90  UpperLimitBoundUnits=deg  UpperLimitStiffness=1e4  UpperLimitStiffnessUnits=N*m/deg  UpperLimitDamping=10  UpperLimitDampingUnits=N*m/(deg/s)  UpperLimitTransitionRegionWidth=0.1  UpperLimitTransitionRegionWidthUnits=deg  PositionTargetSpecify=off  PositionTargetPriority=High  PositionTargetValue=0  PositionTargetValueUnits=deg  VelocityTargetSpecify=off  VelocityTargetPriority=High  VelocityTargetValue=0  VelocityTargetValueUnits=deg/s
  Rigid Transform1 : sm_lib/Frames and Transforms/Rigid Transform  TranslationMethod=Cartesian  TranslationStandardOffset=0  TranslationStandardOffsetUnits=mm  TranslationStandardAxis=+Z  TranslationCartesianOffset=[0 0 0]  TranslationCartesianOffsetUnits=mm  TranslationROffset=0  TranslationROffsetUnits=m  TranslationZOffset=0  TranslationZOffsetUnits=m  TranslationThetaOffset=0  TranslationThetaOffsetUnits=deg  RotationMethod=StandardAxis  RotationAngleUnits=deg  RotationStandardAxis=+X  RotationAngle=0  RotationArbitraryAxis=[0 0 1]  FollAlignAxisA=+X  BaseAlignAxisA=+Y  FollAlignAxisB=+Y  BaseAlignAxisB=+Z  RotationSequenceAxes=FollowerAxes  RotationSequence=XYX  RotationSequenceAngles=[0 0 0]  RotationSequenceAnglesUnits=deg  RotationMatrix=[1 0 0; 0 1 0; 0 0 1]  Quaternion=[1 0 0 0]
  Rigid Transform11 : sm_lib/Frames and Transforms/Rigid Transform  TranslationMethod=Cartesian  TranslationStandardOffset=0  TranslationStandardOffsetUnits=mm  TranslationStandardAxis=+Z  TranslationCartesianOffset=[0 0 0]  TranslationCartesianOffsetUnits=mm  TranslationROffset=0  TranslationROffsetUnits=m  TranslationZOffset=0  TranslationZOffsetUnits=m  TranslationThetaOffset=0  TranslationThetaOffsetUnits=deg  RotationMethod=StandardAxis  RotationAngleUnits=deg  RotationStandardAxis=+Z  RotationAngle=180  RotationArbitraryAxis=[0 0 1]  FollAlignAxisA=+X  BaseAlignAxisA=+Y  FollAlignAxisB=+Y  BaseAlignAxisB=+Z  RotationSequenceAxes=FollowerAxes  RotationSequence=XYX  RotationSequenceAngles=[0 0 0]  RotationSequenceAnglesUnits=deg  RotationMatrix=[1 0 0; 0 1 0; 0 0 1]  Quaternion=[1 0 0 0]
  Simulink-PS Converter1 : nesl_utility/Simulink-PS Converter  PhysicalDomain=network_engine_domain  SubClassName=ps_input  LeftPortType=input  RightPortType=output  PseudoPeriodic=off  Frequencies=[]  NoiseDistribution=none  NoiseParameters=[]  Unit=1  AffineConversion=off  FilteringAndDerivatives=filter  SimscapeFilterOrder=2  InputFilterTimeConstant=0.001  UdotUserProvided=0
  To Workspace1 : ToWorkspace  VariableName=left_motor2  SampleTime=-1
      settings: Save2DSignal=2-D array (concatenate along first dimension)
  Transform Sensor3 : sm_lib/Frames and Transforms/Transform Sensor  MeasurementFrame=NonRotatingFollower  RotationSequence=XYX  SenseAngle=off  SenseAxis=off  SenseQ=off  SenseR=off  SenseRotationSequence=off  SenseOmegaX=off  SenseOmegaY=off  SenseOmegaZ=off  SenseQDot=off  SenseRDot=off  SenseRotationSequenceDot=off  SenseAlphaX=off  SenseAlphaY=off  SenseAlphaZ=off  SenseQDDot=off  SenseRDDot=off  SenseX=on  SenseY=on  SenseZ=on  SenseRad=off  SenseAzim=off  SenseDist=off  SenseInc=off  SenseXDot=off  SenseYDot=off  SenseZDot=off  SenseRadDot=off  SenseAzimDot=off  SenseDistDot=off  SenseIncDot=off  SenseXDDot=off  SenseYDDot=off  SenseZDDot=off  SenseRadDDot=off  SenseAzimDDot=off  SenseDistDDot=off  SenseIncDDot=off
  To Motor 1 : PMIOPort  Side=Left
  To Motor 3 : PMIOPort  Port=2  Side=Right
  World Frame : PMIOPort  Port=3  Side=Right
  tag scope: left_fore_pitch_position=global, left_motor2=global, left_pitch_power=global
  wires:
  PS-Simulink Converter3/1 -> Mux/3  "z"
  Mux/1 -> [left_motor2], To Workspace1/1
  PS-Simulink Converter2/1 -> Mux/2  "y"
  PS-Simulink Converter12/1 -> Mux/1  "x"
  PS-Simulink Converter6/1 -> Product/1
  PS-Simulink Converter/1 -> Product/2
  Product/1 -> [left_pitch_power]
  PS-Simulink Converter4/1 -> [left_fore_pitch_position]
  [left_foreflipper_pitch] -> Simulink-PS Converter1/1
  connections:
  Left Motor 2/LConn1 -- Revolute Joint/RConn1
  To Motor 1/RConn1 -- Rigid Transform1/LConn1
  Rigid Transform11/RConn1 -- Revolute Joint/LConn1
  Rigid Transform1/RConn1 -- Rigid Transform11/LConn1
  Left Motor 2/RConn1 -- Transform Sensor3/RConn1 -- To Motor 3/RConn1
  PS-Simulink Converter2/LConn1 -- Transform Sensor3/RConn3
  PS-Simulink Converter3/LConn1 -- Transform Sensor3/RConn4
  PS-Simulink Converter12/LConn1 -- Transform Sensor3/RConn2
  World Frame/RConn1 -- Transform Sensor3/LConn1
  Simulink-PS Converter1/RConn1 -- Revolute Joint/LConn2
  Revolute Joint/RConn4 -- PS-Simulink Converter/LConn1
  Revolute Joint/RConn3 -- PS-Simulink Converter6/LConn1
  PS-Simulink Converter4/LConn1 -- Revolute Joint/RConn2
